simulink model "main_copy"  (R2023b)
settings: Solver=FixedStepAuto  StartTime=0.0  StopTime=8.5  FixedStep=0.0001  RelTol=1e-3  AbsTol=1e-3  EnableMultiTasking=on
undefined symbols (not defined in the file or in its folder): X, Y, Z
libraries: sm_lib x77, nesl_utility x23, simulink_extras x4, ArmLibrary x2, GripperBaseLibrrary x2, RackLibrary x2, fl_lib x1, LowerLinkLibrary x1, WorkSpaceLibrarry x1
(part 2 of 2)

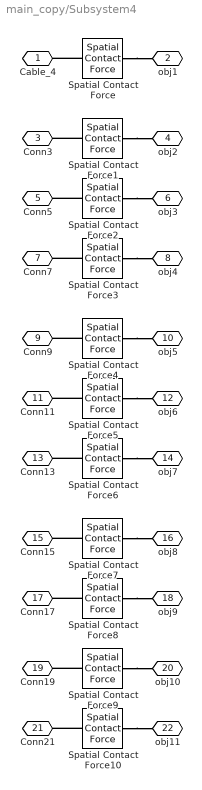
== system main_copy/Subsystem4 ==
  Spatial Contact Force{,1..10} (11 alike) : sm_lib/Forces and Torques/Spatial Contact Force  SenseContactBaseRotation=off  SenseContactBaseTranslation=off  CoefficientOfDynamicFriction=0.3  CoefficientOfStaticFriction=0.5  NormalDamping=1e3  NormalDampingUnits=N/(m/s)  SenseContactSignal=off  NormalStiffness=1e6  NormalStiffnessUnits=N/m  FrictionalCriticalVelocity=1e-3  FrictionalCriticalVelocityUnits=m/s  ZeroCrossDetectContactStartAndEnd=off  SenseContactFollowerRotation=off  SenseContactFollowerTranslation=off  FrictionType=SmoothStickSlip  SenseFrictionalForceMagnitude=off  SenseNormalForceMagnitude=off  NormalForceType=SmoothSpringDamper  SenseNormalVelocity=off  SensePenetrationDepth=off  SenseSeparationDistance=off  SenseTangentialVelocity=off  NormalTransitionRegionWidth=1e-4  NormalTransitionRegionWidthUnits=m
  Cable_4 : PMIOPort  Side=Left
  obj1 : PMIOPort  Port=2  Side=Right
  Conn3 : PMIOPort  Port=3  Side=Left
  obj2 : PMIOPort  Port=4  Side=Right
  Conn5 : PMIOPort  Port=5  Side=Left
  obj3 : PMIOPort  Port=6  Side=Right
  Conn7 : PMIOPort  Port=7  Side=Left
  obj4 : PMIOPort  Port=8  Side=Right
  Conn9 : PMIOPort  Port=9  Side=Left
  obj5 : PMIOPort  Port=10  Side=Right
  Conn11 : PMIOPort  Port=11  Side=Left
  obj6 : PMIOPort  Port=12  Side=Right
  Conn13 : PMIOPort  Port=13  Side=Left
  obj7 : PMIOPort  Port=14  Side=Right
  Conn15 : PMIOPort  Port=15  Side=Left
  obj8 : PMIOPort  Port=16  Side=Right
  Conn17 : PMIOPort  Port=17  Side=Left
  obj9 : PMIOPort  Port=18  Side=Right
  Conn19 : PMIOPort  Port=19  Side=Left
  obj10 : PMIOPort  Port=20  Side=Right
  Conn21 : PMIOPort  Port=21  Side=Left
  obj11 : PMIOPort  Port=22  Side=Right
  connections:
  Spatial Contact Force/RConn1 -- obj1/RConn1
  Spatial Contact Force2/LConn1 -- Conn5/RConn1
  Spatial Contact Force1/RConn1 -- obj2/RConn1
  Spatial Contact Force2/RConn1 -- obj3/RConn1
  Spatial Contact Force1/LConn1 -- Conn3/RConn1
  Spatial Contact Force/LConn1 -- Cable_4/RConn1
  Spatial Contact Force4/RConn1 -- obj5/RConn1
  Spatial Contact Force5/LConn1 -- Conn11/RConn1
  Spatial Contact Force3/LConn1 -- Conn7/RConn1
  Spatial Contact Force4/LConn1 -- Conn9/RConn1
  Spatial Contact Force5/RConn1 -- obj6/RConn1
  Spatial Contact Force3/RConn1 -- obj4/RConn1
  Spatial Contact Force7/RConn1 -- obj8/RConn1
  Spatial Contact Force8/LConn1 -- Conn17/RConn1
  Spatial Contact Force6/LConn1 -- Conn13/RConn1
  Spatial Contact Force7/LConn1 -- Conn15/RConn1
  Spatial Contact Force8/RConn1 -- obj9/RConn1
  Spatial Contact Force6/RConn1 -- obj7/RConn1
  Spatial Contact Force9/LConn1 -- Conn19/RConn1
  Spatial Contact Force10/LConn1 -- Conn21/RConn1
  Spatial Contact Force10/RConn1 -- obj11/RConn1
  Spatial Contact Force9/RConn1 -- obj10/RConn1

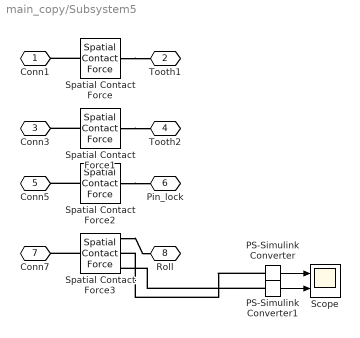
== system main_copy/Subsystem5 ==
  PS-Simulink Converter : nesl_utility/PS-Simulink Converter  PhysicalDomain=network_engine_domain  SubClassName=ps_output  LeftPortType=input  RightPortType=output  PseudoPeriodic=off  Frequencies=[]  VectorFormat=inherit  Unit=N  AffineConversion=off
  PS-Simulink Converter1 : nesl_utility/PS-Simulink Converter  PhysicalDomain=network_engine_domain  SubClassName=ps_output  LeftPortType=input  RightPortType=output  PseudoPeriodic=off  Frequencies=[]  VectorFormat=inherit  Unit=N  AffineConversion=off
  Scope : Scope  NumInputPorts=2
  Spatial Contact Force : sm_lib/Forces and Torques/Spatial Contact Force  SenseContactBaseRotation=off  SenseContactBaseTranslation=off  CoefficientOfDynamicFriction=0.3  CoefficientOfStaticFriction=0.5  NormalDamping=1e3  NormalDampingUnits=N/(m/s)  SenseContactSignal=off  NormalStiffness=1e6  NormalStiffnessUnits=N/m  FrictionalCriticalVelocity=1e-3  FrictionalCriticalVelocityUnits=m/s  ZeroCrossDetectContactStartAndEnd=off  SenseContactFollowerRotation=off  SenseContactFollowerTranslation=off  FrictionType=SmoothStickSlip  SenseFrictionalForceMagnitude=off  SenseNormalForceMagnitude=off  NormalForceType=SmoothSpringDamper  SenseNormalVelocity=off  SensePenetrationDepth=off  SenseSeparationDistance=off  SenseTangentialVelocity=off  NormalTransitionRegionWidth=1e-4  NormalTransitionRegionWidthUnits=m
  Spatial Contact Force1 : sm_lib/Forces and Torques/Spatial Contact Force  SenseContactBaseRotation=off  SenseContactBaseTranslation=off  CoefficientOfDynamicFriction=0.3  CoefficientOfStaticFriction=0.5  NormalDamping=1e3  NormalDampingUnits=N/(m/s)  SenseContactSignal=off  NormalStiffness=1e6  NormalStiffnessUnits=N/m  FrictionalCriticalVelocity=1e-3  FrictionalCriticalVelocityUnits=m/s  ZeroCrossDetectContactStartAndEnd=off  SenseContactFollowerRotation=off  SenseContactFollowerTranslation=off  FrictionType=SmoothStickSlip  SenseFrictionalForceMagnitude=off  SenseNormalForceMagnitude=off  NormalForceType=SmoothSpringDamper  SenseNormalVelocity=off  SensePenetrationDepth=off  SenseSeparationDistance=off  SenseTangentialVelocity=off  NormalTransitionRegionWidth=1e-4  NormalTransitionRegionWidthUnits=m
  Spatial Contact Force2 : sm_lib/Forces and Torques/Spatial Contact Force  SenseContactBaseRotation=off  SenseContactBaseTranslation=off  CoefficientOfDynamicFriction=0.3  CoefficientOfStaticFriction=0.5  NormalDamping=1e3  NormalDampingUnits=N/(m/s)  SenseContactSignal=off  NormalStiffness=1e6  NormalStiffnessUnits=N/m  FrictionalCriticalVelocity=1e-3  FrictionalCriticalVelocityUnits=m/s  ZeroCrossDetectContactStartAndEnd=off  SenseContactFollowerRotation=off  SenseContactFollowerTranslation=off  FrictionType=SmoothStickSlip  SenseFrictionalForceMagnitude=off  SenseNormalForceMagnitude=off  NormalForceType=SmoothSpringDamper  SenseNormalVelocity=off  SensePenetrationDepth=off  SenseSeparationDistance=off  SenseTangentialVelocity=off  NormalTransitionRegionWidth=1e-4  NormalTransitionRegionWidthUnits=m
  Spatial Contact Force3 : sm_lib/Forces and Torques/Spatial Contact Force  SenseContactBaseRotation=off  SenseContactBaseTranslation=off  CoefficientOfDynamicFriction=0.3  CoefficientOfStaticFriction=0.5  NormalDamping=1e3  NormalDampingUnits=N/(m/s)  SenseContactSignal=off  NormalStiffness=1e6  NormalStiffnessUnits=N/m  FrictionalCriticalVelocity=1e-3  FrictionalCriticalVelocityUnits=m/s  ZeroCrossDetectContactStartAndEnd=off  SenseContactFollowerRotation=off  SenseContactFollowerTranslation=off  FrictionType=SmoothStickSlip  SenseFrictionalForceMagnitude=on  SenseNormalForceMagnitude=on  NormalForceType=SmoothSpringDamper  SenseNormalVelocity=off  SensePenetrationDepth=off  SenseSeparationDistance=off  SenseTangentialVelocity=off  NormalTransitionRegionWidth=1e-4  NormalTransitionRegionWidthUnits=m
  Conn1 : PMIOPort  Side=Left
  Tooth1 : PMIOPort  Port=2  Side=Right
  Conn3 : PMIOPort  Port=3  Side=Left
  Tooth2 : PMIOPort  Port=4  Side=Right
  Conn5 : PMIOPort  Port=5  Side=Left
  Pin_lock : PMIOPort  Port=6  Side=Right
  Conn7 : PMIOPort  Port=7  Side=Left
  Roll : PMIOPort  Port=8  Side=Right
  wires:
  PS-Simulink Converter1/1 -> Scope/2
  PS-Simulink Converter/1 -> Scope/1
  connections:
  Spatial Contact Force/LConn1 -- Conn1/RConn1
  Spatial Contact Force1/RConn1 -- Tooth2/RConn1
  Spatial Contact Force/RConn1 -- Tooth1/RConn1
  Spatial Contact Force1/LConn1 -- Conn3/RConn1
  Spatial Contact Force2/LConn1 -- Conn5/RConn1
  Spatial Contact Force3/LConn1 -- Conn7/RConn1
  Spatial Contact Force3/RConn1 -- Roll/RConn1
  Spatial Contact Force2/RConn1 -- Pin_lock/RConn1
  PS-Simulink Converter/LConn1 -- Spatial Contact Force3/RConn2
  PS-Simulink Converter1/LConn1 -- Spatial Contact Force3/RConn3

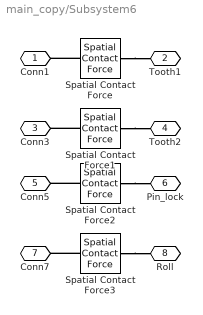
== system main_copy/Subsystem6 ==
  Spatial Contact Force{,1..3} (4 alike) : sm_lib/Forces and Torques/Spatial Contact Force  SenseContactBaseRotation=off  SenseContactBaseTranslation=off  CoefficientOfDynamicFriction=0.3  CoefficientOfStaticFriction=0.5  NormalDamping=1e3  NormalDampingUnits=N/(m/s)  SenseContactSignal=off  NormalStiffness=1e6  NormalStiffnessUnits=N/m  FrictionalCriticalVelocity=1e-3  FrictionalCriticalVelocityUnits=m/s  ZeroCrossDetectContactStartAndEnd=off  SenseContactFollowerRotation=off  SenseContactFollowerTranslation=off  FrictionType=SmoothStickSlip  SenseFrictionalForceMagnitude=off  SenseNormalForceMagnitude=off  NormalForceType=SmoothSpringDamper  SenseNormalVelocity=off  SensePenetrationDepth=off  SenseSeparationDistance=off  SenseTangentialVelocity=off  NormalTransitionRegionWidth=1e-4  NormalTransitionRegionWidthUnits=m
  Conn1 : PMIOPort  Side=Left
  Tooth1 : PMIOPort  Port=2  Side=Right
  Conn3 : PMIOPort  Port=3  Side=Left
  Tooth2 : PMIOPort  Port=4  Side=Right
  Conn5 : PMIOPort  Port=5  Side=Left
  Pin_lock : PMIOPort  Port=6  Side=Right
  Conn7 : PMIOPort  Port=7  Side=Left
  Roll : PMIOPort  Port=8  Side=Right
  connections:
  Spatial Contact Force2/RConn1 -- Pin_lock/RConn1
  Spatial Contact Force3/RConn1 -- Roll/RConn1
  Spatial Contact Force3/LConn1 -- Conn7/RConn1
  Spatial Contact Force2/LConn1 -- Conn5/RConn1
  Spatial Contact Force1/LConn1 -- Conn3/RConn1
  Spatial Contact Force/RConn1 -- Tooth1/RConn1
  Spatial Contact Force1/RConn1 -- Tooth2/RConn1
  Spatial Contact Force/LConn1 -- Conn1/RConn1

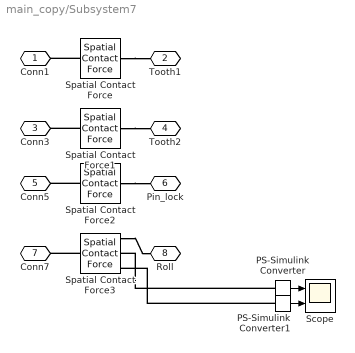
== system main_copy/Subsystem7 ==
  PS-Simulink Converter : nesl_utility/PS-Simulink Converter  PhysicalDomain=network_engine_domain  SubClassName=ps_output  LeftPortType=input  RightPortType=output  PseudoPeriodic=off  Frequencies=[]  VectorFormat=inherit  Unit=N  AffineConversion=off
  PS-Simulink Converter1 : nesl_utility/PS-Simulink Converter  PhysicalDomain=network_engine_domain  SubClassName=ps_output  LeftPortType=input  RightPortType=output  PseudoPeriodic=off  Frequencies=[]  VectorFormat=inherit  Unit=N  AffineConversion=off
  Scope : Scope  NumInputPorts=2
  Spatial Contact Force : sm_lib/Forces and Torques/Spatial Contact Force  SenseContactBaseRotation=off  SenseContactBaseTranslation=off  CoefficientOfDynamicFriction=0.3  CoefficientOfStaticFriction=0.5  NormalDamping=1e3  NormalDampingUnits=N/(m/s)  SenseContactSignal=off  NormalStiffness=1e6  NormalStiffnessUnits=N/m  FrictionalCriticalVelocity=1e-3  FrictionalCriticalVelocityUnits=m/s  ZeroCrossDetectContactStartAndEnd=off  SenseContactFollowerRotation=off  SenseContactFollowerTranslation=off  FrictionType=SmoothStickSlip  SenseFrictionalForceMagnitude=off  SenseNormalForceMagnitude=off  NormalForceType=SmoothSpringDamper  SenseNormalVelocity=off  SensePenetrationDepth=off  SenseSeparationDistance=off  SenseTangentialVelocity=off  NormalTransitionRegionWidth=1e-4  NormalTransitionRegionWidthUnits=m
  Spatial Contact Force1 : sm_lib/Forces and Torques/Spatial Contact Force  SenseContactBaseRotation=off  SenseContactBaseTranslation=off  CoefficientOfDynamicFriction=0.3  CoefficientOfStaticFriction=0.5  NormalDamping=1e3  NormalDampingUnits=N/(m/s)  SenseContactSignal=off  NormalStiffness=1e6  NormalStiffnessUnits=N/m  FrictionalCriticalVelocity=1e-3  FrictionalCriticalVelocityUnits=m/s  ZeroCrossDetectContactStartAndEnd=off  SenseContactFollowerRotation=off  SenseContactFollowerTranslation=off  FrictionType=SmoothStickSlip  SenseFrictionalForceMagnitude=off  SenseNormalForceMagnitude=off  NormalForceType=SmoothSpringDamper  SenseNormalVelocity=off  SensePenetrationDepth=off  SenseSeparationDistance=off  SenseTangentialVelocity=off  NormalTransitionRegionWidth=1e-4  NormalTransitionRegionWidthUnits=m
  Spatial Contact Force2 : sm_lib/Forces and Torques/Spatial Contact Force  SenseContactBaseRotation=off  SenseContactBaseTranslation=off  CoefficientOfDynamicFriction=0.3  CoefficientOfStaticFriction=0.5  NormalDamping=1e3  NormalDampingUnits=N/(m/s)  SenseContactSignal=off  NormalStiffness=1e6  NormalStiffnessUnits=N/m  FrictionalCriticalVelocity=1e-3  FrictionalCriticalVelocityUnits=m/s  ZeroCrossDetectContactStartAndEnd=off  SenseContactFollowerRotation=off  SenseContactFollowerTranslation=off  FrictionType=SmoothStickSlip  SenseFrictionalForceMagnitude=off  SenseNormalForceMagnitude=off  NormalForceType=SmoothSpringDamper  SenseNormalVelocity=off  SensePenetrationDepth=off  SenseSeparationDistance=off  SenseTangentialVelocity=off  NormalTransitionRegionWidth=1e-4  NormalTransitionRegionWidthUnits=m
  Spatial Contact Force3 : sm_lib/Forces and Torques/Spatial Contact Force  SenseContactBaseRotation=off  SenseContactBaseTranslation=off  CoefficientOfDynamicFriction=0.7  CoefficientOfStaticFriction=0.7  NormalDamping=1e3  NormalDampingUnits=N/(m/s)  SenseContactSignal=off  NormalStiffness=1e6  NormalStiffnessUnits=N/m  FrictionalCriticalVelocity=1e-3  FrictionalCriticalVelocityUnits=m/s  ZeroCrossDetectContactStartAndEnd=off  SenseContactFollowerRotation=off  SenseContactFollowerTranslation=off  FrictionType=SmoothStickSlip  SenseFrictionalForceMagnitude=on  SenseNormalForceMagnitude=on  NormalForceType=SmoothSpringDamper  SenseNormalVelocity=off  SensePenetrationDepth=off  SenseSeparationDistance=off  SenseTangentialVelocity=off  NormalTransitionRegionWidth=1e-4  NormalTransitionRegionWidthUnits=m
  Conn1 : PMIOPort  Side=Left
  Tooth1 : PMIOPort  Port=2  Side=Right
  Conn3 : PMIOPort  Port=3  Side=Left
  Tooth2 : PMIOPort  Port=4  Side=Right
  Conn5 : PMIOPort  Port=5  Side=Left
  Pin_lock : PMIOPort  Port=6  Side=Right
  Conn7 : PMIOPort  Port=7  Side=Left
  Roll : PMIOPort  Port=8  Side=Right
  wires:
  PS-Simulink Converter/1 -> Scope/1
  PS-Simulink Converter1/1 -> Scope/2
  connections:
  Spatial Contact Force2/RConn1 -- Pin_lock/RConn1
  Spatial Contact Force3/RConn1 -- Roll/RConn1
  Spatial Contact Force3/LConn1 -- Conn7/RConn1
  Spatial Contact Force2/LConn1 -- Conn5/RConn1
  Spatial Contact Force1/LConn1 -- Conn3/RConn1
  Spatial Contact Force/RConn1 -- Tooth1/RConn1
  Spatial Contact Force1/RConn1 -- Tooth2/RConn1
  Spatial Contact Force/LConn1 -- Conn1/RConn1
  PS-Simulink Converter/LConn1 -- Spatial Contact Force3/RConn2
  PS-Simulink Converter1/LConn1 -- Spatial Contact Force3/RConn3

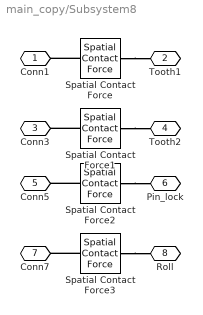
== system main_copy/Subsystem8 ==
  Spatial Contact Force : sm_lib/Forces and Torques/Spatial Contact Force  SenseContactBaseRotation=off  SenseContactBaseTranslation=off  CoefficientOfDynamicFriction=0.3  CoefficientOfStaticFriction=0.5  NormalDamping=1e3  NormalDampingUnits=N/(m/s)  SenseContactSignal=off  NormalStiffness=1e6  NormalStiffnessUnits=N/m  FrictionalCriticalVelocity=1e-3  FrictionalCriticalVelocityUnits=m/s  ZeroCrossDetectContactStartAndEnd=off  SenseContactFollowerRotation=off  SenseContactFollowerTranslation=off  FrictionType=SmoothStickSlip  SenseFrictionalForceMagnitude=off  SenseNormalForceMagnitude=off  NormalForceType=SmoothSpringDamper  SenseNormalVelocity=off  SensePenetrationDepth=off  SenseSeparationDistance=off  SenseTangentialVelocity=off  NormalTransitionRegionWidth=1e-4  NormalTransitionRegionWidthUnits=m
  Spatial Contact Force1 : sm_lib/Forces and Torques/Spatial Contact Force  SenseContactBaseRotation=off  SenseContactBaseTranslation=off  CoefficientOfDynamicFriction=0.3  CoefficientOfStaticFriction=0.5  NormalDamping=1e3  NormalDampingUnits=N/(m/s)  SenseContactSignal=off  NormalStiffness=1e6  NormalStiffnessUnits=N/m  FrictionalCriticalVelocity=1e-3  FrictionalCriticalVelocityUnits=m/s  ZeroCrossDetectContactStartAndEnd=off  SenseContactFollowerRotation=off  SenseContactFollowerTranslation=off  FrictionType=SmoothStickSlip  SenseFrictionalForceMagnitude=off  SenseNormalForceMagnitude=off  NormalForceType=SmoothSpringDamper  SenseNormalVelocity=off  SensePenetrationDepth=off  SenseSeparationDistance=off  SenseTangentialVelocity=off  NormalTransitionRegionWidth=1e-4  NormalTransitionRegionWidthUnits=m
  Spatial Contact Force2 : sm_lib/Forces and Torques/Spatial Contact Force  SenseContactBaseRotation=off  SenseContactBaseTranslation=off  CoefficientOfDynamicFriction=0.3  CoefficientOfStaticFriction=0.5  NormalDamping=1e3  NormalDampingUnits=N/(m/s)  SenseContactSignal=off  NormalStiffness=1e6  NormalStiffnessUnits=N/m  FrictionalCriticalVelocity=1e-3  FrictionalCriticalVelocityUnits=m/s  ZeroCrossDetectContactStartAndEnd=off  SenseContactFollowerRotation=off  SenseContactFollowerTranslation=off  FrictionType=SmoothStickSlip  SenseFrictionalForceMagnitude=off  SenseNormalForceMagnitude=off  NormalForceType=SmoothSpringDamper  SenseNormalVelocity=off  SensePenetrationDepth=off  SenseSeparationDistance=off  SenseTangentialVelocity=off  NormalTransitionRegionWidth=1e-4  NormalTransitionRegionWidthUnits=m
  Spatial Contact Force3 : sm_lib/Forces and Torques/Spatial Contact Force  SenseContactBaseRotation=off  SenseContactBaseTranslation=off  CoefficientOfDynamicFriction=0.7  CoefficientOfStaticFriction=0.7  NormalDamping=1e3  NormalDampingUnits=N/(m/s)  SenseContactSignal=off  NormalStiffness=1e6  NormalStiffnessUnits=N/m  FrictionalCriticalVelocity=1e-3  FrictionalCriticalVelocityUnits=m/s  ZeroCrossDetectContactStartAndEnd=off  SenseContactFollowerRotation=off  SenseContactFollowerTranslation=off  FrictionType=SmoothStickSlip  SenseFrictionalForceMagnitude=off  SenseNormalForceMagnitude=off  NormalForceType=SmoothSpringDamper  SenseNormalVelocity=off  SensePenetrationDepth=off  SenseSeparationDistance=off  SenseTangentialVelocity=off  NormalTransitionRegionWidth=1e-4  NormalTransitionRegionWidthUnits=m
  Conn1 : PMIOPort  Side=Left
  Tooth1 : PMIOPort  Port=2  Side=Right
  Conn3 : PMIOPort  Port=3  Side=Left
  Tooth2 : PMIOPort  Port=4  Side=Right
  Conn5 : PMIOPort  Port=5  Side=Left
  Pin_lock : PMIOPort  Port=6  Side=Right
  Conn7 : PMIOPort  Port=7  Side=Left
  Roll : PMIOPort  Port=8  Side=Right
  connections:
  Spatial Contact Force/LConn1 -- Conn1/RConn1
  Spatial Contact Force1/RConn1 -- Tooth2/RConn1
  Spatial Contact Force/RConn1 -- Tooth1/RConn1
  Spatial Contact Force1/LConn1 -- Conn3/RConn1
  Spatial Contact Force2/LConn1 -- Conn5/RConn1
  Spatial Contact Force3/LConn1 -- Conn7/RConn1
  Spatial Contact Force3/RConn1 -- Roll/RConn1
  Spatial Contact Force2/RConn1 -- Pin_lock/RConn1

== matlab function main_copy/MATLAB Function1 ==
  data: t input; y output
function y = angle(t)
    t_start = 2.7;    % Time when movement begins
    duration = 4.0;   % Transition time in seconds (increase if still too fast)
    
    y_start = -5;
    y_end   = 175;
    
    if t <= t_start
        y = y_start;
    elseif t >= (t_start + duration)
        y = y_end;
    else
        % Normalized time normalized between 0 and 1
        tau = (t - t_start) / duration;
        
        % 5th-order polynomial (smooth 1st and 2nd derivatives)
        s = 6*tau^5 - 15*tau^4 + 10*tau^3;
        
        y = y_start + (y_end - y_start) * s;
    end
end

== matlab function main_copy/MATLAB Function ==
  data: t input; y output; p input
function y = fcn(t, p)
    % =====================================================================
    % CONTROL PARAMETERS
    % =====================================================================
    F_clamp             = -500;    % Target full clamping force (N)
    
    % --- Initial Clamping Parameters ---
    F_approach1         = -0.1;     % Gentle approach force for first clamp (N)
    p_stiffness1        = 0.002;    % Penetration depth for full force (m)
    
    % --- Second Clamping Parameters (Specific to final phase) ---
    F_approach_clamp2   = -0.001;     % Gentle approach force for second clamp (N)
    p_stiffness_clamp2  = 0.0015;   % Penetration depth for second clamp (m)
    
    p_contact           = 0.0;      % Contact position threshold (m)
    
    p_start             = -0.015;   % Position when clamped (m)
    p_target            = 6e-2;     % Target release position (m)
    
    t_release           = 0.5;      % Time to start release (s)
    move_dur            = 0.8;      % Duration of release movement (s)
    
    Kp                  = 150;      % Position tracking gain (N/m)
    Kd_scale            = 0.5;      % Braking scale when overshooting
    
    t_second_clamp      = 7.5;      % Time to re-engage clamping (s)
    % =====================================================================
    p_start2 = 0.06;
    p_target2 =0;
    
    % 1. Initial Clamping Phase
    if t < t_release
        if p < p_contact
            % Gentle approach before contact
            y = F_approach1;
        else
            % Smooth force ramp upon contact based on deflection
            contact_ratio = min(1.0, (p - p_contact) / p_stiffness1);
            y = F_approach1 + (F_clamp - F_approach1) * contact_ratio;
        end
        
    % 2. S-Curve Release & Dynamic Hold Phase
    elseif t >= t_release && t < (t_second_clamp-1.5)
        tau = min(1.0, (t - t_release) / move_dur);
        
        s_curve = tau^3 * (6 * tau^2 - 15 * tau + 10);
        p_ref = p_start + (p_target - p_start) * s_curve;
        
        err = p_ref - p;
        p_start2=p;
        if err >= 0
            y = Kp * err;
        else
            y = Kp * err * (1 + Kd_scale * abs(err));
        end
        
        if tau >= 1.0
            if abs(p_target - p) < 0.003
                y = y * (abs(p_target - p) / 0.003);
            end
        end
        
    % 3. Second Clamping Phase (t >= t_second_clamp)
    elseif t > (t_second_clamp-1.5)  && t <t_second_clamp
        tau = min(1.0, (t - (t_second_clamp-1.5)) / move_dur);
        
        s_curve = tau^3 * (6 * tau^2 - 15 * tau + 10);
        p_ref = p_start2 + (p_target2 - p_start2) * s_curve;
        
        err = p_ref - p;
        
        if err >= 0
            y = Kp * err;
        else
            y = Kp * err * (1 + Kd_scale * abs(err));
        end
        
        if tau >= 1.0
            if abs(p_target2 - p) < 0.003
                y = y * (abs(p_target2 - p) / 0.003);
            end
        end
    else
        y = -500;
    end
end

== matlab function main_copy/MATLAB Function2 ==
  data: t input; y output
function y = angle2(t)
    % --- First Motion Parameters ---
    t_start1  = 1.5;
    duration1 = 1.0;
    y_start1  = 0;
    y_end1    = -13;
    
    % --- Second Motion Parameters ---
    t_start2  = 2.7;
    duration2 = 4.0;
    y_start2  = -13;
    y_end2    =15;
    
    % --- Third Motion Parameters ---
    t_start3  = 7.5;        % Adjust start time as needed
    duration3 = 1.0;        % Adjust duration as needed
    y_start3  = 15;         % Starts at previous end position
    y_end3    = 0;          % Target final position
    
    % --- Motion Trajectory Logic ---
    if t <= t_start1
        % Initial state
        y = y_start1;
        
    elseif t < (t_start1 + duration1)
        % Motion 1: 0 to -13
        tau = (t - t_start1) / duration1;
        s = 6*tau^5 - 15*tau^4 + 10*tau^3;
        y = y_start1 + (y_end1 - y_start1) * s;
        
    elseif t <= t_start2
        % Pause between Motion 1 and Motion 2
        y = y_end1;
        
    elseif t < (t_start2 + duration2)
        % Motion 2: -13 to 10
        tau = (t - t_start2) / duration2;
        s = 6*tau^5 - 15*tau^4 + 10*tau^3;
        y = y_start2 + (y_end2 - y_start2) * s;
        
    elseif t <= t_start3
        % Pause between Motion 2 and Motion 3
        y = y_end2;
        
    elseif t < (t_start3 + duration3)
        % Motion 3: 10 to 0
        tau = (t - t_start3) / duration3;
        s = 6*tau^5 - 15*tau^4 + 10*tau^3;
        y = y_start3 + (y_end3 - y_start3) * s;
        
    else
        % Final state
        y = y_end3;
    end
end

== matlab function main_copy/MATLAB Function3 ==
  data: t input; y output
function y = angle2(t)
    t_start = 2.7;    % Time when movement begins
    duration = 4.0;   % Transition time in seconds (increase if still too fast)
    
    y_start = 13;
    y_end   = -180+13;
    
    if t <= t_start
        y = y_start;
    elseif t >= (t_start + duration)
        y = y_end;
    else
        % Normalized time normalized between 0 and 1
        tau = (t - t_start) / duration;
        
        % 5th-order polynomial (smooth 1st and 2nd derivatives)
        s = 6*tau^5 - 15*tau^4 + 10*tau^3;
        
        y = y_start + (y_end - y_start) * s;
    end
end
